simulink model "Simulation_der_Modelle_neu"  (R2016a)
settings: Solver=VariableStepAuto  StartTime=0.0  StopTime=10.0  RelTol=1e-3
values from neighbouring files (symbols this model uses):
  C1 = zeors(s1*Nu,s1)    [OptimierungMitConstrains.m]    (also in Regerlung_einer_WEA.m = 1)
  C2 = zeors(s1*Nu,s1*Nu)    [OptimierungMitConstrains.m]    (also in Regerlung_einer_WEA.m = [1,0,0,0])
  C3 = [1,0,0,0,0,0 ... (first row only)    [Regerlung_einer_WEA.m]
  C4 = [1,0,0,0,0,0,0,0 ... (first row only)    [Regerlung_einer_WEA.m]
  D1 = zeros(1,3)    [Regerlung_einer_WEA.m]
  D2 = zeros(1,3)    [Regerlung_einer_WEA.m]
  D3 = zeros(3,3)    [Regerlung_einer_WEA.m]
  D4 = zeros(5,3)    [Regerlung_einer_WEA.m]
  T_g_c = [0,0,0,43093.5,43093.5,43093.5]    [Regerlung_einer_WEA.m]
  T_s = 0.05    [Regerlung_einer_WEA.m]
  theta_c = [0,0,0,4,15,22]*pi/180    [Regerlung_einer_WEA.m]
  v_c = [8.0,10.0,11.0,14.0,18.0,25.0]    [Regerlung_einer_WEA.m]    (also in testinterpolation.m = [9,9.5,10,11,14,15,18,25])
undefined symbols (not defined in the file or in its folder): apAC1, apAC2, apAC3, apAC4, apAD1, apAD2, apAD3, apAD4, apBC1, apBC2, apBC3, apBC4, apBD1, apBD2, apBD3, apBD4, i
settings Model: Creator=pasca  LastModifiedBy=pasca

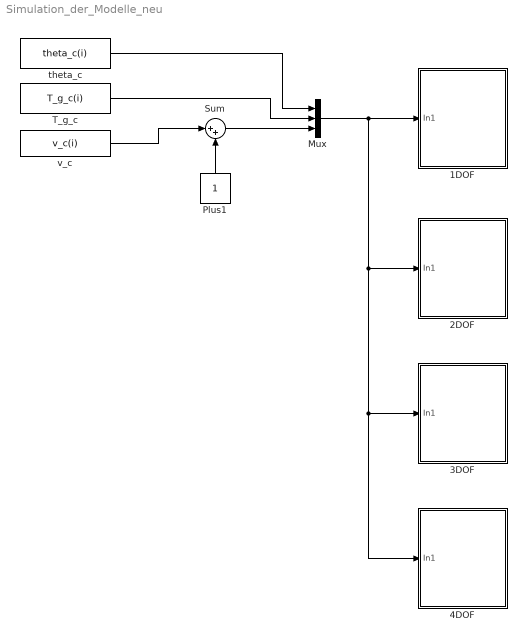
== system Simulation_der_Modelle_neu ==
  1DOF : Subsystem
  2DOF : Subsystem
  3DOF : Subsystem
  4DOF : Subsystem
  Mux : Mux  Inputs=3
  Plus1 : Constant
  Sum : Sum  Inputs=|++
  T_g_c : Constant  Value=T_g_c(i)
  theta_c : Constant  Value=theta_c(i)
  v_c : Constant  Value=v_c(i)
  wires:
  Mux/1 -> 4DOF/1(In1), 3DOF/1(In1), 2DOF/1(In1), 1DOF/1(In1)
  Sum/1 -> Mux/3
  Plus1/1 -> Sum/2
  theta_c/1 -> Mux/1
  T_g_c/1 -> Mux/2
  v_c/1 -> Sum/1

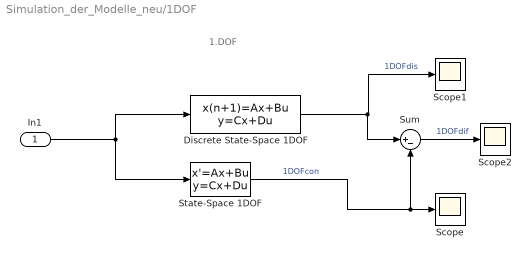
== system Simulation_der_Modelle_neu/1DOF ==
  note: 1.DOF
  In1 : Inport
  Discrete State-Space 1DOF : DiscreteStateSpace  A=apAD1{i}  B=apBD1{i}  C=C1  D=D1  SampleTime=T_s
  Scope : Scope
  Scope1 : Scope
  Scope2 : Scope
  "State-Space 1DOF " : StateSpace  A=apAC1{i}  B=apBC1{i}  C=C1  D=D1  X0=0
  Sum : Sum  Inputs=|+-
  wires:
  Discrete State-Space 1DOF/1 -> Sum/1, Scope1/1  "1DOFdis"
  "State-Space 1DOF "/1 -> Sum/2, Scope/1  "1DOFcon"
  In1/1 -> "State-Space 1DOF "/1, Discrete State-Space 1DOF/1
  Sum/1 -> Scope2/1  "1DOFdif"

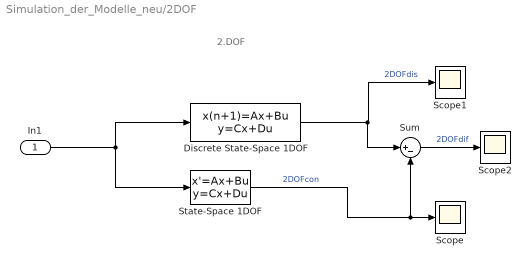
== system Simulation_der_Modelle_neu/2DOF ==
  note: 2.DOF
  In1 : Inport
  Discrete State-Space 1DOF : DiscreteStateSpace  A=apAD2{i}  B=apBD2{i}  C=C2  D=D2  SampleTime=T_s
  Scope : Scope
  Scope1 : Scope
  Scope2 : Scope
  "State-Space 1DOF " : StateSpace  A=apAC2{i}  B=apBC2{i}  C=C2  D=D2  X0=0
  Sum : Sum  Inputs=|+-
  wires:
  Discrete State-Space 1DOF/1 -> Sum/1, Scope1/1  "2DOFdis"
  "State-Space 1DOF "/1 -> Sum/2, Scope/1  "2DOFcon"
  In1/1 -> "State-Space 1DOF "/1, Discrete State-Space 1DOF/1
  Sum/1 -> Scope2/1  "2DOFdif"

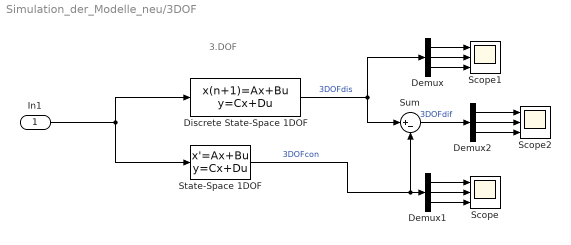
== system Simulation_der_Modelle_neu/3DOF ==
  note: 3.DOF
  In1 : Inport
  Demux : Demux  Outputs=3
  Demux1 : Demux  Outputs=3
  Demux2 : Demux  Outputs=3
  Discrete State-Space 1DOF : DiscreteStateSpace  A=apAD3{i}  B=apBD3{i}  C=C3  D=D3  SampleTime=T_s
  Scope : Scope  NumInputPorts=3
  Scope1 : Scope  NumInputPorts=3
  Scope2 : Scope  NumInputPorts=3
  "State-Space 1DOF " : StateSpace  A=apAC3{i}  B=apBC3{i}  C=C3  D=D3  X0=0
  Sum : Sum  Inputs=|+-
  wires:
  Discrete State-Space 1DOF/1 -> Sum/1, Demux/1  "3DOFdis"
  "State-Space 1DOF "/1 -> Demux1/1, Sum/2  "3DOFcon"
  In1/1 -> "State-Space 1DOF "/1, Discrete State-Space 1DOF/1
  Demux/1 -> Scope1/1
  Sum/1 -> Demux2/1  "3DOFdif"
  Demux/2 -> Scope1/2
  Demux/3 -> Scope1/3
  Demux2/1 -> Scope2/1
  Demux2/2 -> Scope2/2
  Demux2/3 -> Scope2/3
  Demux1/1 -> Scope/1
  Demux1/2 -> Scope/2
  Demux1/3 -> Scope/3

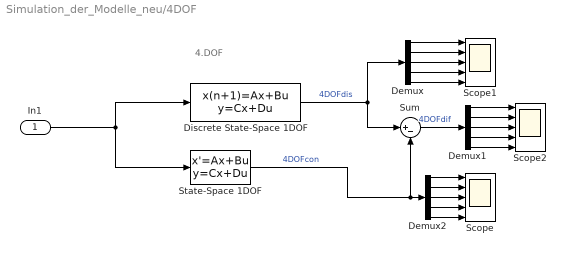
== system Simulation_der_Modelle_neu/4DOF ==
  note: 4.DOF
  In1 : Inport
  Demux : Demux  Outputs=5
  Demux1 : Demux  Outputs=5
  Demux2 : Demux  Outputs=5
  Discrete State-Space 1DOF : DiscreteStateSpace  A=apAD4{i}  B=apBD4{i}  C=C4  D=D4  SampleTime=T_s
  Scope : Scope  NumInputPorts=5
  Scope1 : Scope  NumInputPorts=5
  Scope2 : Scope  NumInputPorts=5
  "State-Space 1DOF " : StateSpace  A=apAC4{i}  B=apBC4{i}  C=C4  D=D4  X0=0
  Sum : Sum  Inputs=|+-
  wires:
  Discrete State-Space 1DOF/1 -> Sum/1, Demux/1  "4DOFdis"
  "State-Space 1DOF "/1 -> Demux2/1, Sum/2  "4DOFcon"
  In1/1 -> "State-Space 1DOF "/1, Discrete State-Space 1DOF/1
  Sum/1 -> Demux1/1  "4DOFdif"
  Demux2/1 -> Scope/1
  Demux2/2 -> Scope/2
  Demux2/3 -> Scope/3
  Demux2/4 -> Scope/4
  Demux2/5 -> Scope/5
  Demux1/1 -> Scope2/1
  Demux1/2 -> Scope2/2
  Demux1/3 -> Scope2/3
  Demux1/4 -> Scope2/4
  Demux1/5 -> Scope2/5
  Demux/1 -> Scope1/1
  Demux/2 -> Scope1/2
  Demux/3 -> Scope1/3
  Demux/4 -> Scope1/4
  Demux/5 -> Scope1/5
